simulink model "traffic_light"  (R2022a)
settings: Solver=FixedStepAuto  StartTime=0.0  StopTime=inf  RelTol=1e-3  EnableMultiTasking=on
settings Model: ExtModeTrigDuration=2  Creator=Amin  LastModifiedBy=Amin
settings OptimizationCC: EnhancedBackFolding=on  PassReuseOutputArgsAs=Individual arguments  ZeroExternalMemoryAtStartup=off  ZeroInternalMemoryAtStartup=off  MaxStackSize=64  OptimizeBlockOrder=speed  DifferentSizesBufferReuse=on  OptimizationCustomize=off  EfficientTunableParamExpr=on
settings DebuggingCC: ParameterTunabilityLossMsg=error
settings HardwareCC: ProdBitPerInt=16  ProdBitPerPointer=16  ProdBitPerSizeT=16  ProdBitPerPtrDiffT=16  ProdLargestAtomicFloat=None  ProdWordSize=8  ProdHWDeviceType=Atmel->AVR
settings SFSimCC: MATLABDynamicMemAlloc=off
settings RTWCC: SystemTargetFile=ert.tlc  HardwareBoard=Arduino Mega 2560  TemplateMakefile=ert_default_tmf  Toolchain=Arduino AVR  BuildConfiguration=Faster Runs
settings CodeAppCC: ForceParamTrailComments=on  IgnoreCustomStorageClasses=off  OperatorAnnotations=on  SimulinkDataObjDesc=on  SFDataObjDesc=on  InsertBlockDesc=on
settings ERTTargetCC: SupportContinuousTime=on  SupportVariableSizeSignals=on  ExtModeTransport=3  ExtModeStaticAlloc=on  ExtModeStaticAllocSize=2048  ExtModeMexFile=ext_xcp  ExtModeIntrfLevel=Level2 - Open
settings ConfigComp: CovEnable=on  RecordCoverage=on  CovModelRefEnable=on

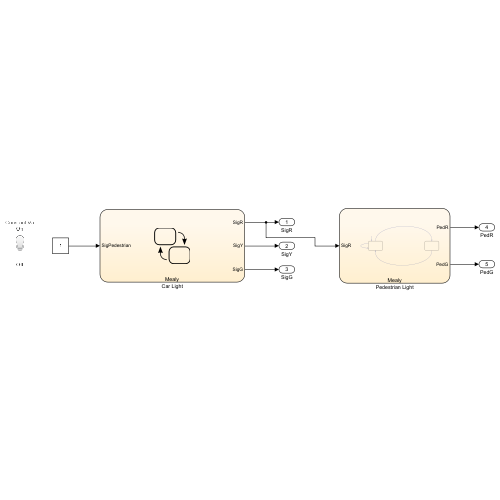
[thumbnail: Simulink's stored preview of the top-level diagram]
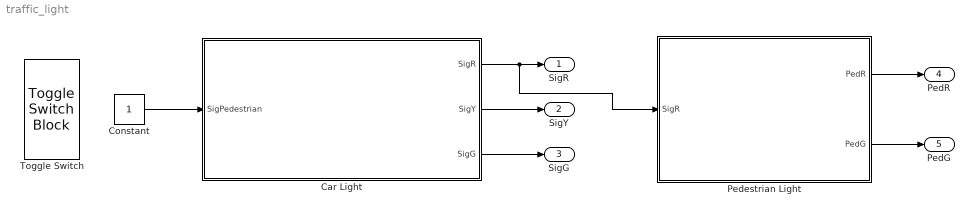
== system traffic_light ==
  Car Light : Stateflow chart  TreatAsAtomicUnit=on
  Constant : Constant
  Pedestrian Light : Stateflow chart  TreatAsAtomicUnit=on
  Toggle Switch : ToggleSwitchBlock
      settings: Values={{'Off', 'On'}, [0 1]}
  SigR : Outport
  SigY : Outport  Port=2
  SigG : Outport  Port=3
  PedR : Outport  Port=4
  PedG : Outport  Port=5
  wires:
  Car Light/1(SigR) -> Pedestrian Light/1(SigR), SigR/1
  Car Light/2(SigY) -> SigY/1
  Car Light/3(SigG) -> SigG/1
  Pedestrian Light/1(PedR) -> PedR/1
  Pedestrian Light/2(PedG) -> PedG/1
  Constant/1 -> Car Light/1(SigPedestrian)

== stateflow chart traffic_light/Pedestrian Light ==
  settings: stateMachineType=MEALY_MACHINE
  state Green
  state Red
  Green -> Red [order 1] : [pcount>=60]{PedR=1;PedG=0}
  (default) -> Green : {pcount=0;PedG=1}
  Green -> Green [order 2] : {pcount=pcount+1;}
  Red -> Green : [SigR==1]{PedG=1;PedR=0;pcount=0;}
  data: SigR input; PedR output; PedG output; pcount local double

== stateflow chart traffic_light/Car Light ==
  settings: stateMachineType=MEALY_MACHINE
  state Green
  state Red
  state Pending
  state Yellow
  Green -> Green [order 3] : [count<60]{count=count+1;}
  Green -> Pending [order 1] : [count<60 && SigPedestrian]{count=count+1;}
  Red -> Green [order 1] : [count>=60]{SigG=1;SigR=0;count=0}
  Green -> Yellow [order 2] : [count>=60&&SigPedestrian]{SigY=1;SigG=0;count=0}
  (default) -> Red : {count=0;SigR=1}
  Pending -> Pending [order 2] : {count=count+1;}
  Red -> Red [order 2] : {count=count+1;}
  Yellow -> Red [order 1] : [count>=5]{SigR=1;SigY=0;count=0}
  Pending -> Yellow [order 1] : [count>=60]{SigY=1;SigG=0;count=0;}
  Yellow -> Yellow [order 2] : {count=count+1;}
  data: count local double; SigPedestrian input; SigR output double; SigY output double; SigG output double
